simulink model "motorbb"  (R2022a)
settings: Solver=VariableStepAuto  StartTime=0.0  StopTime=10.0  RelTol=1e-3
libraries: mbedblockslib x6, simulink x1
settings Model: Creator=Matlab  LastModifiedBy=Matlab

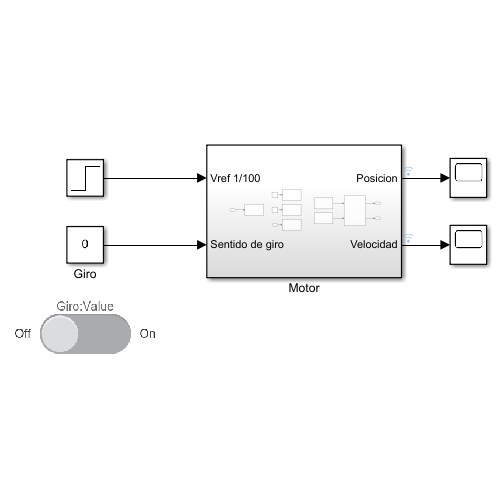
[thumbnail: Simulink's stored preview of the top-level diagram]
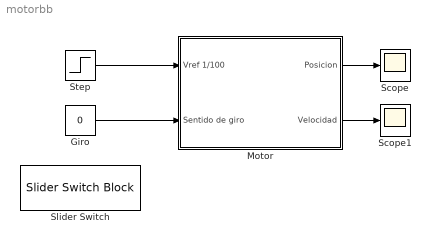
== system motorbb ==
  Giro : Constant  Value=0
  Motor : Subsystem
  Scope : Scope
  Scope1 : Scope
  Slider Switch : SliderSwitchBlock
      settings: Values={{'Off', 'On'}, [0 1]}
  Step : Step  SampleTime=0
  wires:
  Step/1 -> Motor/1(Vref 1/100)
  Giro/1 -> Motor/2(Sentido de giro)
  Motor/1(Posicion) -> Scope/1
  Motor/2(Velocidad) -> Scope1/1

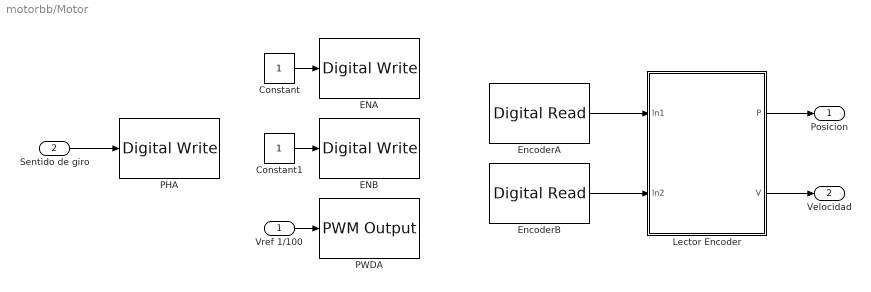
== system motorbb/Motor ==
  Vref 1/100 : Inport
  Sentido de giro : Inport  Port=2
  Constant : Constant
  Constant1 : Constant
  ENA : mbedblockslib/Digital Write  Pin=D2  Direction=output
      settings: SourceProductBaseCode=MICROBIT,NUCLEO,STMICRODIS
  ENB : mbedblockslib/Digital Write  Pin=D11  Direction=output
      settings: SourceProductBaseCode=MICROBIT,NUCLEO,STMICRODIS
  EncoderA : mbedblockslib/Digital Read  Pin=A1  Direction=input  SampleTime=0.1
      settings: SourceProductBaseCode=MICROBIT,NUCLEO,STMICRODIS
  EncoderB : mbedblockslib/Digital Read  Pin=A0  Direction=input  SampleTime=0.1
      settings: SourceProductBaseCode=MICROBIT,NUCLEO,STMICRODIS
  Lector Encoder : Subsystem
  PHA : mbedblockslib/Digital Write  Pin=D5  Direction=output
      settings: SourceProductBaseCode=MICROBIT,NUCLEO,STMICRODIS
  PWDA : mbedblockslib/PWM Output  Pin=D5  EnableInputFrequency=off  InitialFrequency=5000  InitialDutyCycle=0  NotificationType=None
      settings: SourceProductBaseCode=MICROBIT,NUCLEO,STMICRODIS
  Posicion : Outport
  Velocidad : Outport  Port=2
  wires:
  Sentido de giro/1 -> PHA/1
  Vref 1/100/1 -> PWDA/1
  Constant/1 -> ENA/1
  Constant1/1 -> ENB/1
  EncoderA/1 -> Lector Encoder/1(In1)
  EncoderB/1 -> Lector Encoder/2(In2)
  Lector Encoder/2(V) -> Velocidad/1
  Lector Encoder/1(P) -> Posicion/1

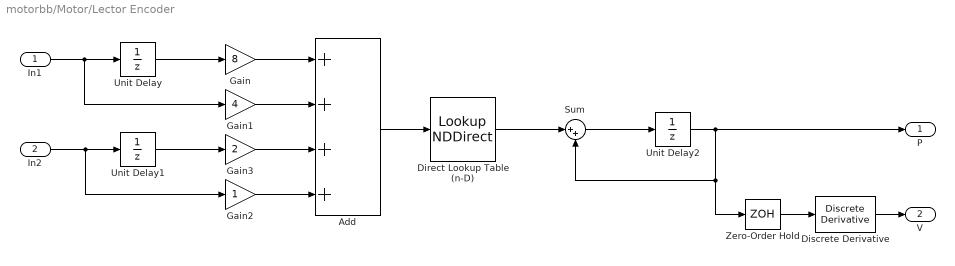
== system motorbb/Motor/Lector Encoder ==
  In1 : Inport
  In2 : Inport  Port=2
  Add : Sum  Inputs=++++  OutDataTypeStr=double
  Direct Lookup Table (n-D) : LookupNDDirect  NumberOfTableDimensions=1  Table=[0, -1, 1, 0, 1, 0, 0, -1, -1, 0, 0, 1, 0, 1, -1, 0]
  Discrete Derivative : simulink/Discrete/Discrete Derivative  gainval=1.0  ICPrevScaledInput=0.0  OutMin=[]  OutMax=[]  OutDataType=fixdt(1, 16)  OutScaling=2^-10  DoSatur=off
  Gain : Gain  Gain=8
  Gain1 : Gain  Gain=4
  Gain2 : Gain
  Gain3 : Gain  Gain=2
  Sum : Sum  Inputs=|++
  Unit Delay : UnitDelay  SampleTime=-1  HasFrameUpgradeWarning=on
  Unit Delay1 : UnitDelay  SampleTime=-1  HasFrameUpgradeWarning=on
  Unit Delay2 : UnitDelay  SampleTime=-1  HasFrameUpgradeWarning=on
  Zero-Order Hold : ZeroOrderHold  SampleTime=0.01
  P : Outport
  V : Outport  Port=2
  wires:
  In1/1 -> Unit Delay/1, Gain1/1
  Unit Delay/1 -> Gain/1
  In2/1 -> Gain2/1, Unit Delay1/1
  Unit Delay1/1 -> Gain3/1
  Gain/1 -> Add/1
  Gain1/1 -> Add/2
  Gain3/1 -> Add/3
  Gain2/1 -> Add/4
  Add/1 -> Direct Lookup Table (n-D)/1
  Sum/1 -> Unit Delay2/1
  Direct Lookup Table (n-D)/1 -> Sum/1
  Unit Delay2/1 -> P/1, Sum/2, Zero-Order Hold/1
  Zero-Order Hold/1 -> Discrete Derivative/1
  Discrete Derivative/1 -> V/1
